simulink model "abEPMAFPLL_compare_discrete_integrations"  (R2020b)
settings: Solver=FixedStepAuto  StartTime=0.0  StopTime=36.72  FixedStep=Ts  MaxStep=1e-5  RelTol=1e-3
values from neighbouring files (symbols this model uses):
  N = T_MAF/Ts    (= 200)    [maf_filter.m]
  Ts = 1/fs    (= 0.0001)    [maf_filter.m]
undefined symbols (not defined in the file or in its folder): A_frq_step, A_phase_step, DiscIntNeverNeededParam, f_rad, k_phi, ki, kp, t_frq_step, t_phase_step, V_g, var_noise
libraries: simulink x8, bach_library x3
settings Model: Creator=Martin  LastModifiedBy=Kasper Laustsen
settings DataIOCC: ExternalInput=tt1, tt2, tt3, tt4, tt5, tt6  LoadExternalInput=on

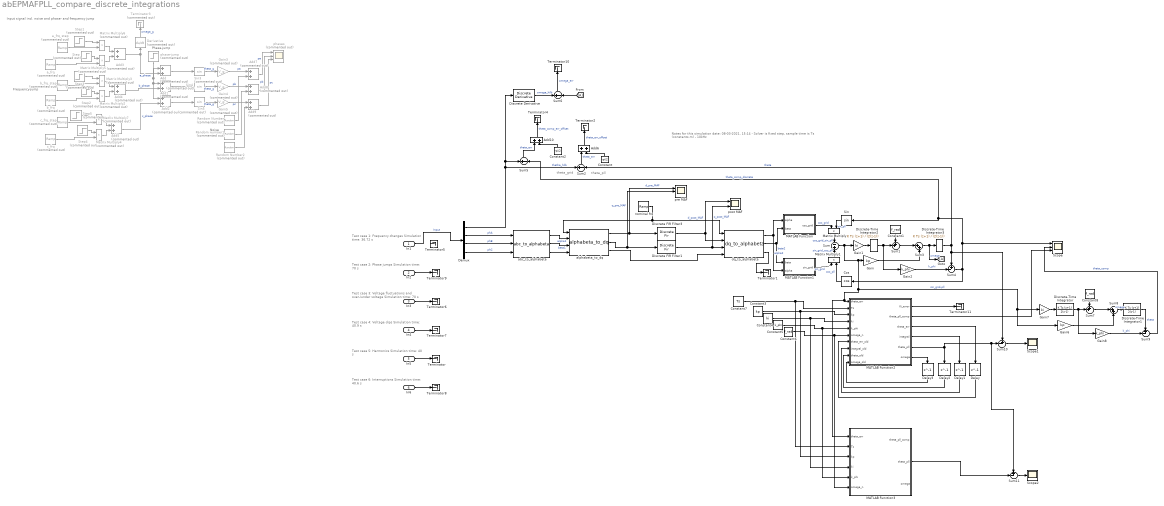
== system abEPMAFPLL_compare_discrete_integrations ==
  note: Input signal incl. noise and phase- and frequency jump
  note: Notes for this simulation
      |
      | date: 08-03-2021, 15:14
      | - Solver is fixed step, sample time is Ts (constants.m) - 10kHz
  note: Noise
  note: Phase-jump
  note: theta_grid
  note: theta_pll
  note: Frequency-jump
  note: Test case 2: Phase jumps
      | Simulation time: 70 s
  note: Test case 1: Frequency changes
      | Simulation time: 36.72 s
  note: Test case 3: Voltage fluctuations
      | and over-/under voltage
      | Simulation time: 70 s
  note: Test case 4: Voltage dips
      | Simulation time: 40.9 s
  note: Test case 5: Harmonics
      | Simulation time: 40 s
  note: Test case 6: Interruptions
      | Simulation time: 40.6 s
  In1 : Inport  PortDimensions=4
  In2 : Inport  Port=2  PortDimensions=4
  In3 : Inport  Port=3  PortDimensions=4
  In4 : Inport  Port=4  PortDimensions=4
  In5 : Inport  Port=5  PortDimensions=4
  In6 : Inport  Port=6  PortDimensions=4
  Add{,1..5,7..9} (9 alike) : Sum  Commented=on
  Add10 : Sum
  Add6 : Sum
  Constant : Constant  Value=-pi/2
  Constant1 : Constant  Value=f_rad
  Constant2 : Constant  Value=-pi/2
  Constant3 : Constant  Value=kp
  Constant4 : Constant  Value=ki
  Constant5 : Constant  Value=k_phi
  Constant6 : Constant  Value=f_rad
  Constant7 : Constant  Value=Ts
  Constant8 : Constant  Value=f_rad
  Cos : Trigonometry  Operator=cos
  Delay{,1..3} (4 alike) : Delay  DelayLength=1
  Demux : Demux
  Derivative : Derivative  Commented=on
  Discrete Derivative : simulink/Discrete/Discrete Derivative  gainval=1.0  ICPrevScaledInput=0.0  OutMin=[]  OutMax=[]  OutDataType=fixdt(1, 16)  OutScaling=2^-10  DoSatur=off
  Discrete FIR Filter1 : DiscreteFir  Coefficients=[ones(1,N).*1/N]
  Discrete FIR Filter3 : DiscreteFir  Coefficients=[ones(1,N).*1/N]
  Discrete-Time Integrator{,1..3} (4 alike) : DiscreteIntegrator  IntegratorMethod=Integration: Trapezoidal  SampleTime=-1  ICPrevOutput=DiscIntNeverNeededParam  ICPrevScaledInput=DiscIntNeverNeededParam
  Gain : Gain  Gain=kp
  Gain1 : Gain  Gain=ki
  Gain2 : Gain  Gain=k_phi
  Gain3 : Gain  Commented=on  Gain=V_g
  Gain4 : Gain  Commented=on  Gain=V_g
  Gain5 : Gain  Commented=on  Gain=V_g
  Gain6 : Gain  Gain=kp
  Gain7 : Gain  Gain=ki
  Gain8 : Gain  Gain=k_phi
  MATLAB Function : MATLAB Function  TreatAsAtomicUnit=on
  MATLAB Function1 : MATLAB Function  TreatAsAtomicUnit=on
  MATLAB Function2 : MATLAB Function  TreatAsAtomicUnit=on
  MATLAB Function3 : MATLAB Function  TreatAsAtomicUnit=on
  Matrix Multiply : Product
  Matrix Multiply1 : Product
  Matrix Multiply{2..7} (6 alike) : Product  Commented=on
  Random Number : RandomNumber  Commented=on  Variance=var_noise
  Random Number1 : RandomNumber  Commented=on  Variance=var_noise  Seed=1
  Random Number2 : RandomNumber  Commented=on  Variance=var_noise  Seed=2
  Scope : Scope  NumInputPorts=3
  Scope1 : Scope
  Scope2 : Scope
  Sin : Trigonometry
  Sin3 : Trigonometry  Commented=on
  Sin4 : Trigonometry  Commented=on
  Sin5 : Trigonometry  Commented=on
  Step : Step  Commented=on  Time=t_frq_step  Before=1  After=0  SampleTime=0
  Step1 : Step  Commented=on  Time=t_frq_step  SampleTime=0
  Step2 : Step  Commented=on  Time=t_frq_step  Before=1  After=0  SampleTime=0
  Step3 : Step  Commented=on  Time=t_frq_step  SampleTime=0
  Step4 : Step  Commented=on  Time=t_frq_step  Before=1  After=0  SampleTime=0
  Step5 : Step  Commented=on  Time=t_frq_step  SampleTime=0
  Sum : Sum  Inputs=-|+
  Sum1 : Sum  Inputs=++|
  Sum{4,9..11} (4 alike) : Sum  Inputs=+-|
  Sum2 : Sum  Inputs=+|-
  Sum3 : Sum  Inputs=|++
  Sum5 : Sum  Inputs=+|-
  Sum6 : Sum  Inputs=+|-
  Sum7 : Sum  Inputs=++|
  Sum8 : Sum  Inputs=|++
  Terminator{,1..2,4..11} (11 alike) : Terminator
  Terminator3 : Terminator  Commented=on
  a_frq : simulink/Sources/Ramp  Commented=on  slope=f_rad  start=0  InitialOutput=0
  a_frq_step : simulink/Sources/Ramp  Commented=on  slope=f_rad*A_frq_step  start=t_frq_step  InitialOutput=t_frq_step*f_rad
  abc_to_alphabeta : bach_library/abc_to_alphabeta  SystemSampleTime=-1  VariantActivationTime=update diagram  Latency=0  AutoFrameSizeCalculation=off
  alphabeta_to_dq : bach_library/alphabeta_to_dq  SystemSampleTime=-1  VariantActivationTime=update diagram  Latency=0  AutoFrameSizeCalculation=off
  b_frq : simulink/Sources/Ramp  Commented=on  slope=f_rad  start=0  InitialOutput=-pi*2/3
  b_frq_step : simulink/Sources/Ramp  Commented=on  slope=f_rad*A_frq_step  start=t_frq_step  InitialOutput=t_frq_step*f_rad-pi*2/3
  c_frq : simulink/Sources/Ramp  Commented=on  slope=f_rad  start=0  InitialOutput=pi*2/3
  c_frq_step : simulink/Sources/Ramp  Commented=on  slope=f_rad*A_frq_step  start=t_frq_step  InitialOutput=t_frq_step*f_rad+pi*2/3
  dq_to_alphabeta : bach_library/dq_to_alphabeta  SystemSampleTime=-1  VariantActivationTime=update diagram  Latency=0  AutoFrameSizeCalculation=off
  nominal frq : simulink/Sources/Ramp  slope=f_rad  start=0  InitialOutput=0
  phase-jump : Step  Commented=on  Time=t_phase_step  After=A_phase_step  SampleTime=0
  phases : Scope  Commented=on  NumInputPorts=3
  post MAF : Scope  NumInputPorts=2
  pre MAF : Scope  NumInputPorts=3
  wires:
  Derivative/1 -> Terminator3/1  "omega_g"
  Step2/1 -> Matrix Multiply2/1
  MATLAB Function/1(cos_grid) -> Matrix Multiply/1  "cos_grid"
  Constant/1 -> Add6/2
  Step/1 -> Matrix Multiply5/1
  Sin5/1 -> Gain5/1  "theta_g"
  Sin3/1 -> Gain3/1  "theta_g"
  Step1/1 -> Matrix Multiply6/1
  a_frq/1 -> Matrix Multiply5/2
  Step4/1 -> Matrix Multiply4/1
  Matrix Multiply2/1 -> Add4/2
  Matrix Multiply7/1 -> Add5/1
  Matrix Multiply6/1 -> Add3/1
  a_frq_step/1 -> Matrix Multiply6/2
  Add6/1 -> Terminator2/1  "theta_err_offset"
  Sum2/1 -> Add6/1  "theta_err"
  Sin/1 -> Matrix Multiply/2  "sin_pll"
  Add1/1 -> Sin4/1
  phase-jump/1 -> Add/1, Add2/1, Add1/1
  Matrix Multiply4/1 -> Add5/2
  Add4/1 -> Add1/2  "b_phase"
  Add9/1 -> phases/3  "pc"
  Add5/1 -> Add2/2  "c_phase"
  Cos/1 -> Matrix Multiply1/2  "cos_pll"
  Add7/1 -> phases/1  "pa"
  Matrix Multiply/1 -> Sum/1  "cos_grid_sin_pll"
  Add8/1 -> phases/2  "pb"
  Add/1 -> Sin3/1
  Random Number/1 -> Add7/2
  Step3/1 -> Matrix Multiply3/1
  Add2/1 -> Sin5/1
  Gain3/1 -> Add7/1  "pa"
  c_frq/1 -> Matrix Multiply4/2
  Matrix Multiply5/1 -> Add3/2
  Add3/1 -> Add/2, Derivative/1  "a_phase"
  Matrix Multiply3/1 -> Add4/1
  Sin4/1 -> Gain4/1  "theta_g"
  MATLAB Function1/1(sin_grid) -> Matrix Multiply1/1  "sin_grid"
  Matrix Multiply1/1 -> Sum/2  "sin_grid_cos_pll"
  Random Number1/1 -> Add8/2
  b_frq_step/1 -> Matrix Multiply3/2
  Random Number2/1 -> Add9/2
  b_frq/1 -> Matrix Multiply2/2
  c_frq_step/1 -> Matrix Multiply7/2
  Gain5/1 -> Add9/1  "pc"
  Gain4/1 -> Add8/1  "pb"
  Step5/1 -> Matrix Multiply7/1
  Gain1/1 -> Discrete-Time Integrator2/1
  Gain/1 -> Sum3/2
  Discrete-Time Integrator2/1 -> Sum1/2, Gain2/1
  Discrete-Time Integrator3/1 -> Sum2/2, Sum10/1, Sum4/1  "theta"
  Gain2/1 -> Sum4/2  "k_phi"
  Sum4/1 -> Cos/1, Scope/1, Sum5/2, Sin/1  "theta_comp_discrete"
  abc_to_alphabeta/3 -> alphabeta_to_dq/4
  dq_to_alphabeta/1 -> MATLAB Function/1(alpha), MATLAB Function1/2(alpha)  "alpha2"
  dq_to_alphabeta/2 -> MATLAB Function1/1(beta), MATLAB Function/2(beta)  "beta2"
  nominal frq/1 -> dq_to_alphabeta/1, alphabeta_to_dq/1
  abc_to_alphabeta/1 -> alphabeta_to_dq/2  "alpha1"
  abc_to_alphabeta/2 -> alphabeta_to_dq/3  "beta1"
  alphabeta_to_dq/2 -> Discrete FIR Filter1/1, pre MAF/2  "q_pre_MAF"
  alphabeta_to_dq/1 -> pre MAF/1, Discrete FIR Filter3/1  "d_pre_MAF"
  Discrete FIR Filter3/1 -> post MAF/1, dq_to_alphabeta/2  "d_post_MAF"
  Discrete FIR Filter1/1 -> post MAF/2, dq_to_alphabeta/3  "q_post_MAF"
  alphabeta_to_dq/3 -> dq_to_alphabeta/4
  Sum1/1 -> Sum3/1
  Constant1/1 -> Sum1/1
  Sum3/1 -> Discrete-Time Integrator3/1, [A]  "omega"
  dq_to_alphabeta/3 -> Terminator1/1
  Add10/1 -> Terminator4/1  "theta_comp_err_offset"
  Sum5/1 -> Add10/1  "theta_err"
  Constant2/1 -> Add10/2
  Demux/2 -> abc_to_alphabeta/1  "phA"
  Demux/4 -> abc_to_alphabeta/3  "phC"
  Demux/3 -> abc_to_alphabeta/2  "phB"
  Demux/1 -> Sum2/1, Discrete Derivative/1, Sum5/1  "thetha_hilb"
  Discrete Derivative/1 -> Sum6/1  "omega_hilb"
  [A] -> Sum6/2
  Sum6/1 -> Terminator10/1  "omega_err"
  In1/1 -> Demux/1  "Input"
  In2/1 -> Terminator9/1
  In3/1 -> Terminator6/1
  In4/1 -> Terminator7/1
  In5/1 -> Terminator/1
  In6/1 -> Terminator8/1
  MATLAB Function2/4(integral) -> Delay1/1
  MATLAB Function2/3(theta_err) -> Delay/1
  MATLAB Function2/6(omega) -> Delay3/1
  MATLAB Function2/5(theta_pll) -> Delay2/1, Sum11/1, Sum10/2
  Constant3/1 -> MATLAB Function3/3(kp), MATLAB Function2/3(kp)
  Constant4/1 -> MATLAB Function3/4(ki), MATLAB Function2/4(ki)
  Constant5/1 -> MATLAB Function3/5(k_phi), MATLAB Function2/5(k_phi)
  Constant6/1 -> MATLAB Function3/6(omega_n), MATLAB Function2/6(omega_n)
  Delay/1 -> MATLAB Function2/7(theta_err_old)
  Delay1/1 -> MATLAB Function2/8(integral_old)
  Delay2/1 -> MATLAB Function2/9(theta_old)
  Delay3/1 -> MATLAB Function2/10(omega_old)
  Constant7/1 -> MATLAB Function3/2(Ts), MATLAB Function2/2(Ts)
  MATLAB Function2/1(Ki_error) -> Terminator11/1
  Gain6/1 -> Sum8/2
  Gain8/1 -> Sum9/2  "k_phi"
  Constant8/1 -> Sum7/1
  Sum7/1 -> Sum8/1
  Sum8/1 -> Discrete-Time Integrator1/1  "omega"
  Discrete-Time Integrator1/1 -> Sum9/1  "theta"
  Discrete-Time Integrator/1 -> Sum7/2, Gain8/1
  Gain7/1 -> Discrete-Time Integrator/1
  Sum/1 -> Gain1/1, Gain7/1, Gain6/1, MATLAB Function3/1(theta_err), MATLAB Function2/1("theta_err "), Gain/1  "sin_grid-pll"
  Sum9/1 -> Scope/2  "theta_comp"
  MATLAB Function2/2(theta_pll_comp) -> Scope/3
  Sum10/1 -> Scope1/1
  Sum11/1 -> Scope2/1
  MATLAB Function3/2(theta_pll) -> Sum11/2

== matlab function abEPMAFPLL_compare_discrete_integrations/MATLAB Function1 ==
  data: beta input; alpha input; sin_grid output
function sin_grid = sin_grid(beta, alpha)

sin_grid = beta/sqrt(alpha^2+beta^2);

== matlab function abEPMAFPLL_compare_discrete_integrations/MATLAB Function ==
  data: alpha input; cos_grid output; beta input
function cos_grid = cos_grid(alpha, beta)

cos_grid = alpha/sqrt(alpha^2+beta^2);

== matlab function abEPMAFPLL_compare_discrete_integrations/MATLAB Function2 ==
  data: Ki_error output; theta_err input; Ts input; theta_pll_comp output; theta_err output; integral output; kp input; ki input; k_phi input; omega_n input; theta_err_old input; integral_old input; theta_old input; omega_old input; theta_pll output; omega output
function [Ki_error, theta_pll_comp, theta_err, integral, theta_pll, omega]  = fcn(theta_err, Ts, kp, ki, k_phi, omega_n, theta_err_old, integral_old, theta_old, omega_old)

% persistent theta_old integral_old;
Ki_error = ki*theta_err;
% integral = Ki_error*0.5 + ki*theta_err_old*0.5 + integral_old;
integral = ki*(theta_err*0.5 + theta_err_old*0.5)*Ts + integral_old;
omega = theta_err*kp + integral + omega_n; 

theta_pll = (omega*0.5 + omega_old*0.5)*Ts + theta_old; 
theta_pll_comp = theta_pll - (omega - omega_n - theta_err*kp)*k_phi;

% integral_old = integral
% omega_old = omega;
% theta_err_old = theta_err

== matlab function abEPMAFPLL_compare_discrete_integrations/MATLAB Function3 ==
  data: theta_err input; Ts input; theta_pll_comp output; theta_pll output; kp input; ki input; k_phi input; omega_n input; omega output
function [theta_pll_comp, theta_pll, omega]  = fcn(theta_err, Ts, kp, ki, k_phi, omega_n)

persistent theta_err_old integral_old theta_old omega_old;
if isempty(theta_err_old)
        theta_err_old = 0;
end
if isempty(integral_old)
        integral_old = 0;
end
if isempty(theta_old)
        theta_old = 0;
end
if isempty(omega_old)
        omega_old = 0;
end

% Ki_error = ki*theta_err;
% integral = Ki_error*0.5 + ki*theta_err_old*0.5 + integral_old;
integral = ki*(theta_err*0.5 + theta_err_old*0.5)*Ts + integral_old;
omega = theta_err*kp + integral + omega_n; 

theta_pll = (omega*0.5 + omega_old*0.5)*Ts + theta_old; 
theta_pll_comp = theta_pll - (omega - omega_n - theta_err*kp)*k_phi;

theta_err_old = theta_err;
integral_old = integral;
theta_old = theta_pll;
omega_old = omega;

% integral_old = integral
% omega_old = omega;
% theta_err_old = theta_err
